simulink model "BLDC_DQ"  (R2020a)
settings: Solver=VariableStepAuto  StartTime=0.0  StopTime=10.0  RelTol=1e-3
settings Model: Creator=enzoe  LastModifiedBy=enzoe

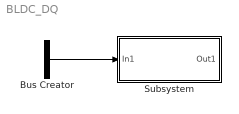
== system BLDC_DQ ==
  Bus Creator : BusCreator  Inputs=2
  Subsystem : Subsystem
  wires:
  Bus Creator/1 -> Subsystem/1(In1)
  ? -> Bus Creator/1  "Vd"
  ? -> Bus Creator/2  "Vq"

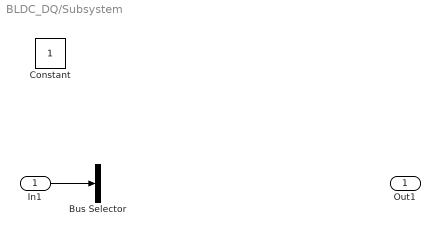
== system BLDC_DQ/Subsystem ==
  In1 : Inport
  Bus Selector : BusSelector  OutputSignals=signal1,signal2
  Constant : Constant
  Out1 : Outport
  wires:
  In1/1 -> Bus Selector/1
